simulink model "closed_loop_PID"  (R2023a)
settings: Solver=FixedStepAuto  StartTime=0.0  StopTime=20  FixedStep=0.01  RelTol=1e-3  EnableMultiTasking=on
values from neighbouring files (symbols this model uses):
  CAf = 1.0    (= 1)    [A1_Task8_param_consts.m]    (also in find_steady_state.m)
  Cp = 0.239    [A1_Task8_param_consts.m]    (also in find_steady_state.m)
  dHr = -5e4    (= -50000)    [A1_Task8_param_consts.m]    (also in find_steady_state.m)
  ER = 8750    [A1_Task8_param_consts.m]    (also in find_steady_state.m)
  k0 = 6.379829e+10    (= 63798290000)    [A1_Task8_param_consts.m]    (also in find_steady_state.m)
  Ki = Kp/Ti    (= 3272.72727273)    [A1_Task8_param_consts.m]
  Kp = Ku/2.2    (= 54.5454545455)    [A1_Task8_param_consts.m]
  q = 100    [A1_Task8_param_consts.m]    (also in find_steady_state.m)
  rho = 1000    [A1_Task8_param_consts.m]    (also in find_steady_state.m)
  Tf = 350    [A1_Task8_param_consts.m]    (also in find_steady_state.m)
  UA = 5e4    (= 50000)    [A1_Task8_param_consts.m]    (also in find_steady_state.m)
  V = 100    [A1_Task8_param_consts.m]    (also in find_steady_state.m)
libraries: slpidlib x1
settings Model: Creator=xiong  LastModifiedBy=xiong

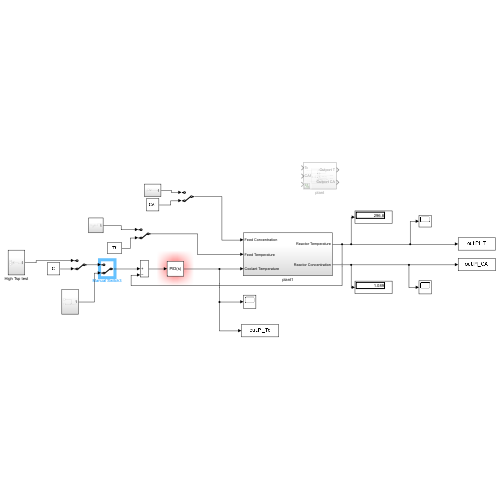
[thumbnail: Simulink's stored preview of the top-level diagram]
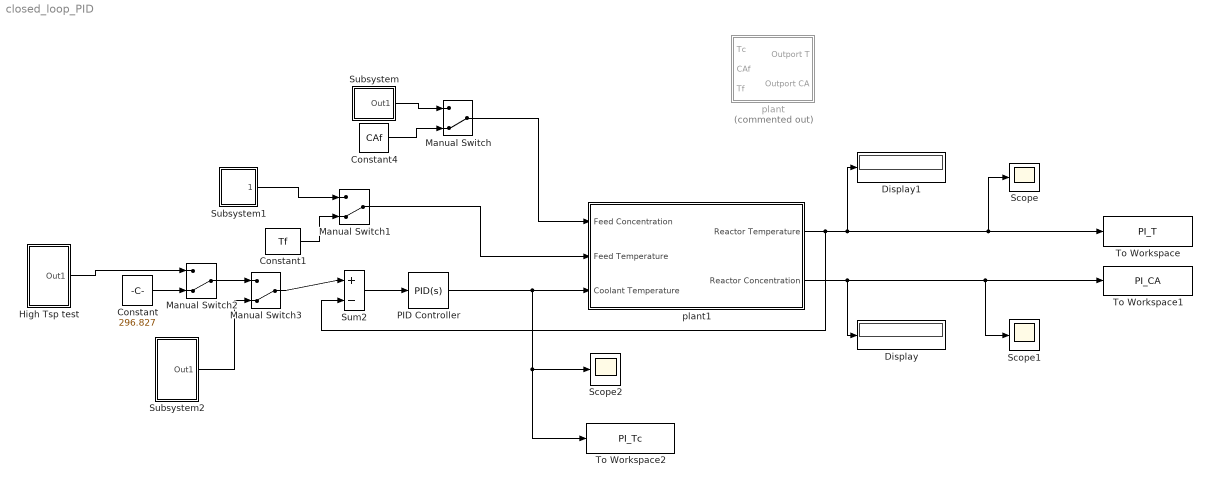
== system closed_loop_PID ==
  Constant : Constant  Value=296.827
  Constant1 : Constant  Value=Tf
  Constant4 : Constant  Value=CAf
  Display : Display
  Display1 : Display
  High Tsp test : Subsystem
  Manual Switch{,1..3} (4 alike) : ManualSwitch  CurrentSetting=0
  PID Controller : slpidlib/PID Controller  Controller=PID  Form=Parallel  TimeDomain=Continuous-time  UseExternalTs=off  SampleTime=-1  IntegratorMethod=Forward Euler  FilterMethod=Forward Euler  ControllerParametersSource=internal  P=Kp  I=Ki  UseKiTs=off  D=0  N=0  UseFilter=on  TunerSelectOption=Transfer Function Based (PID Tuner App)  InitialConditionSource=internal  InitialConditionForIntegrator=0  InitialConditionForFilter=0  DifferentiatorICPrevScaledInput=0  ExternalReset=none  TrackingMode=off  Kt=1  LimitOutput=off  SatLimitsSource=internal  UpperSaturationLimit=inf  LowerSaturationLimit=-inf  LinearizeAsGain=on  AntiWindupMode=none  Kb=1  LimitIntegrator=off  UpperIntegratorSaturationLimit=inf  LowerIntegratorSaturationLimit=-inf  POutMin=[]  POutMax=[]  IOutMin=[]  IOutMax=[]  DOutMin=[]  DOutMax=[]  NOutMin=[]  NOutMax=[]  SumOutMin=[]  SumOutMax=[]  SaturationOutMin=[]  SaturationOutMax=[]  PParamMin=[]  PParamMax=[]  IParamMin=[]  IParamMax=[]  DParamMin=[]  DParamMax=[]  NParamMin=[]  NParamMax=[]  KbParamMin=[]  KbParamMax=[]  KtParamMin=[]  KtParamMax=[]  KbOutMin=[]  KbOutMax=[]  KtOutMin=[]  KtOutMax=[]  IntegratorOutMin=[]  IntegratorOutMax=[]  FilterOutMin=[]  FilterOutMax=[]  SumI1OutMin=[]  SumI1OutMax=[]  SumI2OutMin=[]  SumI2OutMax=[]  SumI3OutMin=[]  SumI3OutMax=[]  SumI4OutMin=[]  SumI4OutMax=[]  SumDOutMin=[]  SumDOutMax=[]  DifferentiatorOutMin=[]  DifferentiatorOutMax=[]  FilterDiffOutCoefMin=[]  FilterDiffOutCoefMax=[]  ReciprocalOutMin=[]  ReciprocalOutMax=[]  SumDenOutMin=[]  SumDenOutMax=[]  SumNumOutMin=[]  SumNumOutMax=[]  DivideOutMin=[]  DivideOutMax=[]  UdiffTsProdOutMin=[]  UdiffTsProdOutMax=[]  NTsProdOutMin=[]  NTsProdOutMax=[]  UintegralTsProdOutMin=[]  UintegralTsProdOutMax=[]  UngainTsProdOutMin=[]  UngainTsProdOutMax=[]  ClampingZeroOutDataTypeStr=Inherit: Inherit via back propagation  ClampingZeroOutMin=[]  ClampingZeroOutMax=[]  FilterDenConstantOutDataTypeStr=Inherit: Inherit via back propagation  FilterDenConstantOutMin=[]  FilterDenConstantOutMax=[]  PCopyOutDataTypeStr=Inherit: Inherit via back propagation  PCopyOutMin=[]  PCopyOutMax=[]  NCopyOutDataTypeStr=Inherit: Inherit via back propagation  NCopyOutMin=[]  NCopyOutMax=[]  IntegratorContinuousStateAttributes=''  IntegratorStateMustResolveToSignalObject=off  IntegratorRTWStateStorageClass=Auto  FilterContinuousStateAttributes=''  FilterStateMustResolveToSignalObject=off  FilterRTWStateStorageClass=Auto  ParallelPVariant=InternalParameters  IdealPVariant=Disabled  IVariant=InternalParameters  DVariant=InternalParameters  IntegratorVariant=Continuous  SatVariant=Disabled  AWVariant=Passthrough  PCopyVariant=Disabled  TRVariant=Disabled  FdbkBlocksVariant=Forward  IdealPFdbkVariant=Disabled  SatFdbkVariant=Disabled  DerivativeFilterVariant=ContFilter  NVariant=InternalParameters  NCopyVariant=Disabled  FilterICVariant=InternalICsFilter  IntegratorICVariant=InternalICs  ExternalResetVariant=Disabled  TRSumVariant=Passthrough  SumFdbkVariant=Disabled  SumVariant=Sum_PID  TsampFilterVariant=InternalTs  TsampNgainVariant=Passthrough  TsampIntegralVariant=Disabled_SignalSpec  ExternalSaturationOutDataTypeStr=Inherit: Same as second input
  Scope : Scope
  Scope1 : Scope
  Scope2 : Scope
  Subsystem : Subsystem
  Subsystem1 : Subsystem
  Subsystem2 : Subsystem
  Sum2 : Sum  Inputs=|+-
  To Workspace : ToWorkspace  VariableName=PI_T  SaveFormat=Timeseries  SampleTime=-1
  To Workspace1 : ToWorkspace  VariableName=PI_CA  SaveFormat=Timeseries  SampleTime=-1
  To Workspace2 : ToWorkspace  VariableName=PI_Tc  SaveFormat=Timeseries  SampleTime=-1
  plant : Subsystem  Commented=on
  plant1 : Subsystem
  wires:
  plant1/1(Reactor Temperature) -> Sum2/2, Display1/1, Scope/1, To Workspace/1
  plant1/2(Reactor Concentration) -> Display/1, Scope1/1, To Workspace1/1
  Sum2/1 -> PID Controller/1
  Subsystem/1(Out1) -> Manual Switch/1
  Constant4/1 -> Manual Switch/2
  Manual Switch/1 -> plant1/1(Feed Concentration)
  Subsystem1/1(Out1) -> Manual Switch1/1
  Constant1/1 -> Manual Switch1/2
  PID Controller/1 -> To Workspace2/1, Scope2/1, plant1/3(Coolant Temperature)
  Subsystem2/1(Out1) -> Manual Switch3/2
  Constant/1 -> Manual Switch2/2
  Manual Switch2/1 -> Manual Switch3/1
  Manual Switch1/1 -> plant1/2(Feed Temperature)
  Manual Switch3/1 -> Sum2/1
  High Tsp test/1(Out1) -> Manual Switch2/1

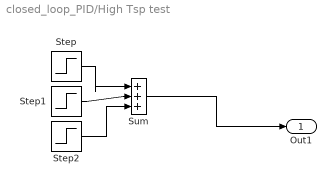
== system closed_loop_PID/High Tsp test ==
  Step : Step  Time=8  Before=400  After=450  SampleTime=0
  Step1 : Step  Time=12  After=50  SampleTime=0
  Step2 : Step  Time=16  After=50  SampleTime=0
  Sum : Sum  Inputs=|+++
  Out1 : Outport
  wires:
  Step1/1 -> Sum/2
  Step2/1 -> Sum/3
  Step/1 -> Sum/1
  Sum/1 -> Out1/1

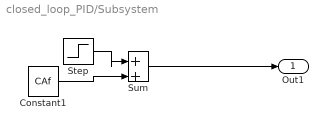
== system closed_loop_PID/Subsystem ==
  Constant1 : Constant  Value=CAf
  Step : Step  Time=2  After=0.1  SampleTime=0
  Sum : Sum  Inputs=|++
  Out1 : Outport
  wires:
  Constant1/1 -> Sum/2
  Step/1 -> Sum/1
  Sum/1 -> Out1/1

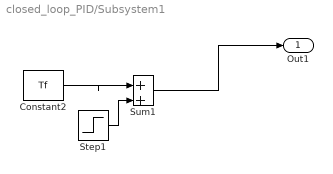
== system closed_loop_PID/Subsystem1 ==
  Constant2 : Constant  Value=Tf
  Step1 : Step  Time=4  After=10  SampleTime=0
  Sum1 : Sum  Inputs=|++
  Out1 : Outport
  wires:
  Sum1/1 -> Out1/1
  Constant2/1 -> Sum1/1
  Step1/1 -> Sum1/2

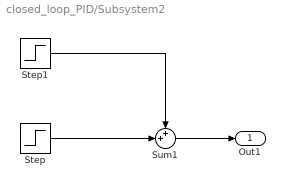
== system closed_loop_PID/Subsystem2 ==
  Step : Step  Time=8  Before=300  After=320  SampleTime=0
  Step1 : Step  Time=12  After=-40  SampleTime=0
  Sum1 : Sum  Inputs=++|
  Out1 : Outport
  wires:
  Step/1 -> Sum1/2
  Step1/1 -> Sum1/1
  Sum1/1 -> Out1/1

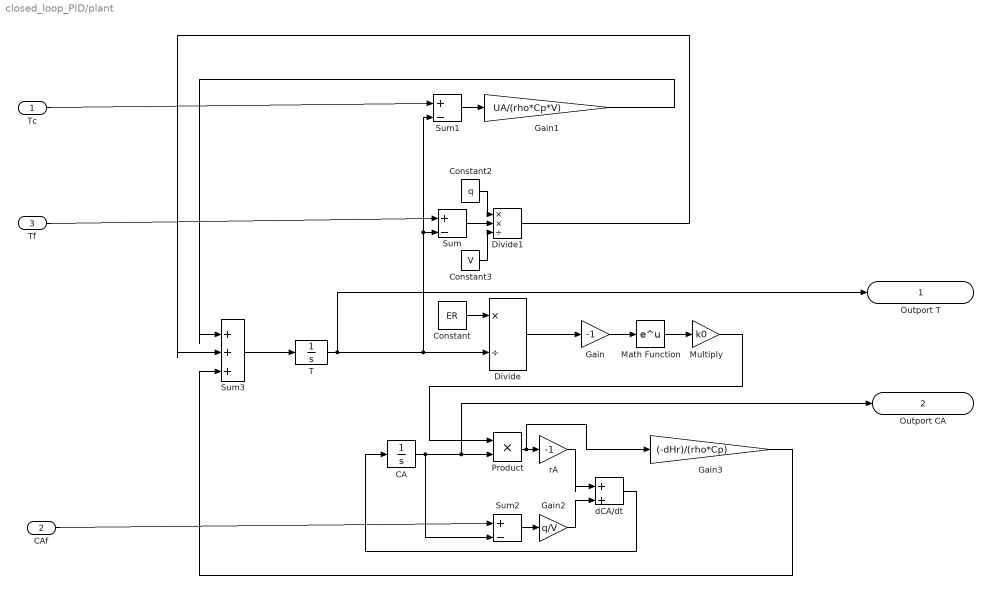
== system closed_loop_PID/plant ==
  Tc : Inport
  CAf : Inport  Port=2
  Tf : Inport  Port=3
  CA : Integrator  InitialCondition=0.5  LimitOutput=on  LowerSaturationLimit=0
  Constant : Constant  Value=ER
  Constant2 : Constant  Value=q
  Constant3 : Constant  Value=V
  Divide : Product  Inputs=*/
  Divide1 : Product  Inputs=**/
  Gain : Gain  Gain=-1
  Gain1 : Gain  Gain=UA/(rho*Cp*V)
  Gain2 : Gain  Gain=q/V
  Gain3 : Gain  Gain=(-dHr)/(rho*Cp)
  Math Function : Math
  Multiply : Gain  Gain=k0
  Product : Product
  Sum : Sum  Inputs=|+-
  Sum1 : Sum  Inputs=|+-
  Sum2 : Sum  Inputs=|+-
  Sum3 : Sum  Inputs=|+++
  T : Integrator  Tag=T  InitialCondition=305  LimitOutput=on  UpperSaturationLimit=800  LowerSaturationLimit=0  ContinuousStateAttributes='T'
  dCA/dt : Sum  Inputs=|++
  rA : Gain  Gain=-1
  Outport T : Outport
  Outport CA : Outport  Port=2
  wires:
  Multiply/1 -> Product/1
  Sum/1 -> Divide1/2
  T/1 -> Outport T/1, Sum1/2, Sum/2, Divide/2
  Gain/1 -> Math Function/1
  Divide1/1 -> Sum3/2
  Product/1 -> Gain3/1, rA/1
  Gain1/1 -> Sum3/1
  CA/1 -> Outport CA/1, Product/2, Sum2/2
  CAf/1 -> Sum2/1
  Divide/1 -> Gain/1
  Constant/1 -> Divide/1
  rA/1 -> dCA/dt/1
  Tc/1 -> Sum1/1
  Sum2/1 -> Gain2/1
  Constant3/1 -> Divide1/3
  dCA/dt/1 -> CA/1
  Tf/1 -> Sum/1
  Math Function/1 -> Multiply/1
  Constant2/1 -> Divide1/1
  Sum3/1 -> T/1
  Gain3/1 -> Sum3/3
  Gain2/1 -> dCA/dt/2
  Sum1/1 -> Gain1/1

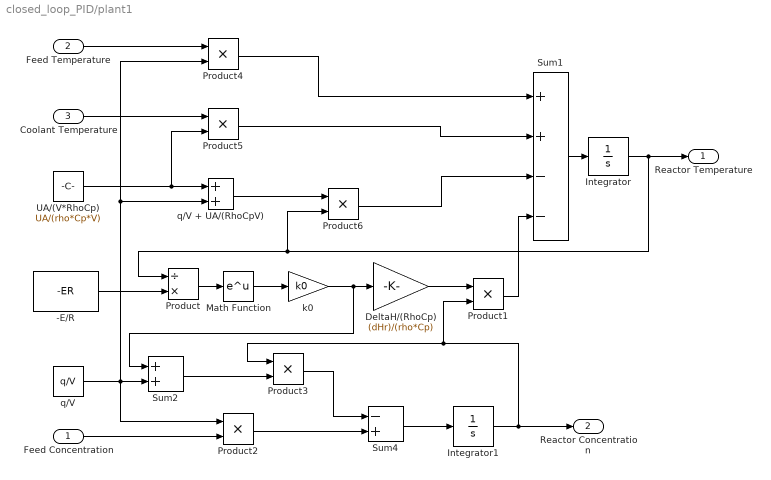
== system closed_loop_PID/plant1 ==
  Feed Concentration : Inport
  Feed Temperature : Inport  Port=2
  Coolant Temperature : Inport  Port=3
  -E/R : Constant  Value=-ER
  DeltaH/(RhoCp) : Gain  Gain=(dHr)/(rho*Cp)  SaturateOnIntegerOverflow=on  OutDataTypeStr=Inherit: Same as input  ParamDataTypeStr=Inherit: Same as input
  Integrator : Integrator  InitialCondition=305  LimitOutput=on  LowerSaturationLimit=0
  Integrator1 : Integrator  InitialCondition=0.5  LimitOutput=on  LowerSaturationLimit=0
  Math Function : Math  SignedPower=on
  Product : Product  Inputs=/*  InputSameDT=on  RndMeth=Zero  SaturateOnIntegerOverflow=on  OutDataTypeStr=Inherit: Same as first input
  Product1 : Product  InputSameDT=on  RndMeth=Zero  SaturateOnIntegerOverflow=on  OutDataTypeStr=Inherit: Same as first input
  Product{2,4..6} (4 alike) : Product
  Product3 : Product  InputSameDT=on  RndMeth=Zero  SaturateOnIntegerOverflow=on  OutDataTypeStr=Inherit: Same as first input
  Sum1 : Sum  Inputs=++--  InputSameDT=on  SaturateOnIntegerOverflow=on  OutDataTypeStr=Inherit: Same as first input
  Sum2 : Sum  InputSameDT=on  SaturateOnIntegerOverflow=on  OutDataTypeStr=Inherit: Same as first input
  Sum4 : Sum  Inputs=-+  InputSameDT=on  SaturateOnIntegerOverflow=on  OutDataTypeStr=Inherit: Same as first input
  UA/(V*RhoCp) : Constant  Value=UA/(rho*Cp*V)
  k0 : Gain  Gain=k0  SaturateOnIntegerOverflow=on  OutDataTypeStr=Inherit: Same as input  ParamDataTypeStr=Inherit: Same as input
  q/V : Constant  Value=q/V
  q/V + UA/(RhoCpV) : Sum
  Reactor Temperature : Outport
  Reactor Concentration : Outport  Port=2
  wires:
  Product4/1 -> Sum1/1
  Sum1/1 -> Integrator/1
  Integrator/1 -> Product6/2, Product/1, Reactor Temperature/1
  Product5/1 -> Sum1/2
  Product6/1 -> Sum1/3
  Product/1 -> Math Function/1
  Math Function/1 -> k0/1
  DeltaH/(RhoCp)/1 -> Product1/1
  Product1/1 -> Sum1/4
  k0/1 -> DeltaH/(RhoCp)/1, Sum2/1
  -E/R/1 -> Product/2
  Product3/1 -> Sum4/1
  Sum4/1 -> Integrator1/1
  Integrator1/1 -> Product1/2, Product3/1, Reactor Concentration/1
  q/V/1 -> Product2/1, Sum2/2, Product4/2, q/V + UA/(RhoCpV)/2
  Product2/1 -> Sum4/2
  Feed Temperature/1 -> Product4/1
  Feed Concentration/1 -> Product2/2
  Coolant Temperature/1 -> Product5/1
  Sum2/1 -> Product3/2
  UA/(V*RhoCp)/1 -> Product5/2, q/V + UA/(RhoCpV)/1
  q/V + UA/(RhoCpV)/1 -> Product6/1
